simulink subsystem "Thrust_Forces_Moments"  (R2025b)
settings: Solver=VariableStepAuto  StartTime=0.0  StopTime=10.0  RelTol=1e-3
undefined symbols (not defined in the file): NumberOfEngines, phi_T, psi_T, R_n, Rho0, T_Max0, x_T_in, y_T_in, y_T_out, z_T_in, z_T_out
settings Model: Creator=cdriggs  LastModifiedBy=Ky Bui

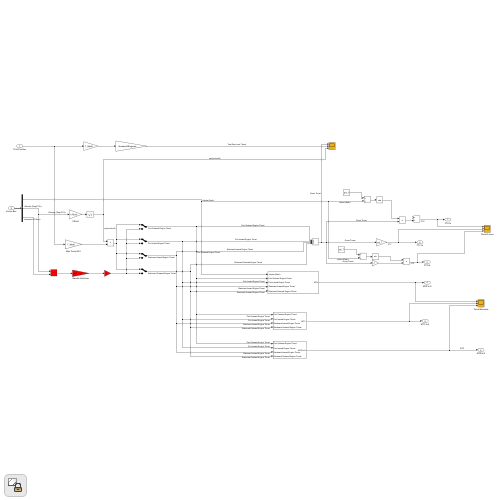
[thumbnail: Simulink's stored preview of the top-level diagram]
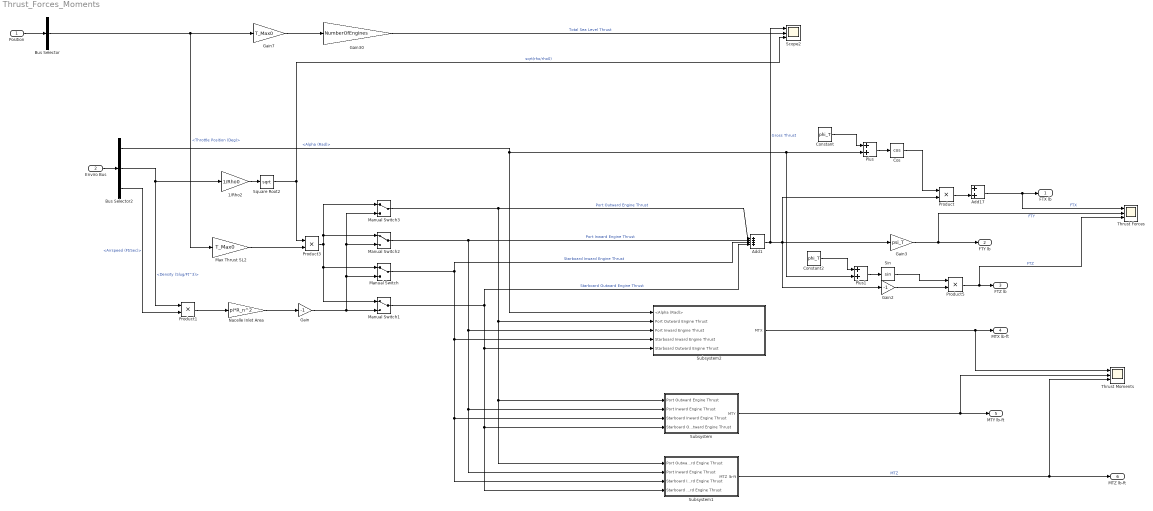
== system Thrust_Forces_Moments ==
  Position : Inport
  Enviro Bus : Inport  Port=2
  1/Rho2 : Gain  Gain=1/Rho0
  Add1 : Sum  Inputs=++++
  Add17 : Sum
  Bus Selector : BusSelector  OutputSignals=Throttle Position (Deg)
  Bus Selector2 : BusSelector  OutputSignals=Aero angles.Alpha (Rad),Density (Slug/Ft^3),Airspeed (Ft/Sec)
  Constant : Constant  Value=phi_T
  Constant2 : Constant  Value=phi_T
  Cos : Trigonometry  Operator=cos
  Gain : Gain  Gain=-1
  Gain2 : Gain  Gain=-1
  Gain3 : Gain  Gain=psi_T
  Gain30 : Gain  Gain=NumberOfEngines
  Gain7 : Gain  Gain=T_Max0
  Manual Switch{,1..3} (4 alike) : ManualSwitch
  Max Thrust SL2 : Gain  Gain=T_Max0
  Nacelle Inlet Area : Gain  Gain=pi*R_n^2
  Plus : Sum
  Plus1 : Sum
  Product{,1,3,5} (4 alike) : Product
  Scope2 : Scope  NumInputPorts=3
      settings: ActiveDisplayYMinimum=62520.103031363164  ActiveDisplayYMaximum=69799.500358108562  DataLoggingVariableName=ScopeData11
  Sin : Trigonometry
  Square Root2 : Sqrt
  Subsystem : Subsystem
  Subsystem1 : Subsystem
  Subsystem2 : Subsystem
  Thrust Forces : Scope  NumInputPorts=3
      settings: ActiveDisplayYMinimum=-15674.497725695244  ActiveDisplayYMaximum=81341.997508548971  DataLoggingVariableName=ScopeData4
  Thrust Moments : Scope  NumInputPorts=3
      settings: ActiveDisplayYMinimum=-5421.00895528758  ActiveDisplayYMaximum=48789.080597588152  DataLoggingVariableName=ScopeData5
  FTX lb : Outport
  FTY lb : Outport  Port=2
  FTZ lb : Outport  Port=3
  MTX lb-ft : Outport  Port=4
  MTY lb-ft : Outport  Port=5
  MTZ lb-ft : Outport  Port=6
  wires:
  Bus Selector2/1 -> Plus1/2, Plus/2, Subsystem2/1(<Alpha (Rad)>)  "<Alpha (Rad)>"
  Bus Selector2/2 -> 1/Rho2/1, Product1/1  "<Density (Slug/Ft^3)>"
  Add1/1 -> Scope2/1, Gain3/1, Product/2, Gain2/1  "Gross Thrust"
  Manual Switch3/1 -> Add1/1, Subsystem/1(Port Outward Engine Thrust), Subsystem1/1(Port Outward Engine Thrust), Subsystem2/2(Port Outward Engine Thrust)  "Port Outward Engine Thrust"
  Product/1 -> Add17/2
  Product3/1 -> Manual Switch3/1, Manual Switch2/1, Manual Switch1/1, Manual Switch/1
  Gain2/1 -> Product5/2
  Cos/1 -> Product/1
  Subsystem1/1(MTZ lb-ft) -> Thrust Moments/3, MTZ lb-ft/1  "MTZ"
  Constant/1 -> Plus/1
  Gain3/1 -> FTY lb/1, Thrust Forces/2  "FTY"
  Manual Switch/1 -> Subsystem2/4(Starboard Inward Engine Thrust), Subsystem/3(Starboard Inward Engine Thrust), Subsystem1/3(Starboard Inward Engine Thrust), Add1/3  "Starboard Inward Engine Thrust"
  Manual Switch2/1 -> Add1/2, Subsystem/2(Port Inward Engine Thrust), Subsystem1/2(Port Inward Engine Thrust), Subsystem2/3(Port Inward Engine Thrust)  "Port Inward Engine Thrust"
  Enviro Bus/1 -> Bus Selector2/1
  Constant2/1 -> Plus1/1
  Max Thrust SL2/1 -> Product3/2
  Manual Switch1/1 -> Subsystem2/5(Starboard Outward Engine Thrust), Subsystem/4(Starboard Outward Engine Thrust), Subsystem1/4(Starboard Outward Engine Thrust), Add1/4  "Starboard Outward Engine Thrust"
  Sin/1 -> Product5/1
  1/Rho2/1 -> Square Root2/1
  Add17/1 -> FTX lb/1, Thrust Forces/1  "FTX"
  Gain30/1 -> Scope2/2  "Total Sea Level Thrust"
  Plus1/1 -> Sin/1
  Square Root2/1 -> Product3/1, Scope2/3  "sqrt(rho/rho0)"
  Gain7/1 -> Gain30/1
  Product5/1 -> FTZ lb/1, Thrust Forces/3  "FTZ"
  Plus/1 -> Cos/1
  Subsystem/1(MTY) -> Thrust Moments/2, MTY lb-ft/1
  Subsystem2/1(MTX) -> MTX lb-ft/1, Thrust Moments/1
  Bus Selector2/3 -> Product1/2  "<Airspeed (Ft/Sec)>"
  Nacelle Inlet Area/1 -> Gain/1
  Product1/1 -> Nacelle Inlet Area/1
  Gain/1 -> Manual Switch3/2, Manual Switch2/2, Manual Switch/2, Manual Switch1/2
  Position/1 -> Bus Selector/1
  Bus Selector/1 -> Gain7/1, Max Thrust SL2/1  "<Throttle Position (Deg)>"

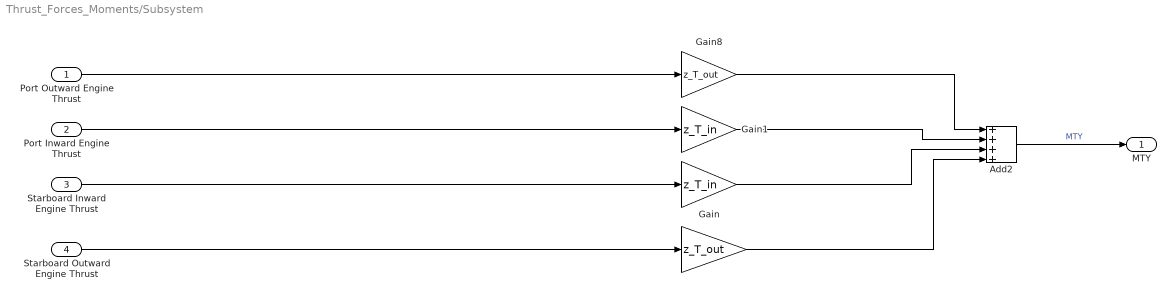
== system Thrust_Forces_Moments/Subsystem ==
  Port Outward Engine Thrust : Inport
  Port Inward Engine Thrust : Inport  Port=2
  Starboard Inward Engine Thrust : Inport  Port=3
  Starboard Outward Engine Thrust : Inport  Port=4
  " " : Gain  Gain=z_T_out
  Add2 : Sum  Inputs=++++
  Gain : Gain  Gain=z_T_in
  Gain1 : Gain  Gain=z_T_in
  Gain8 : Gain  Gain=z_T_out
  MTY : Outport
  wires:
  Port Outward Engine Thrust/1 -> Gain8/1
  Starboard Outward Engine Thrust/1 -> " "/1
  " "/1 -> Add2/4
  Starboard Inward Engine Thrust/1 -> Gain/1
  Port Inward Engine Thrust/1 -> Gain1/1
  Gain1/1 -> Add2/2
  Add2/1 -> MTY/1  "MTY"
  Gain/1 -> Add2/3
  Gain8/1 -> Add2/1

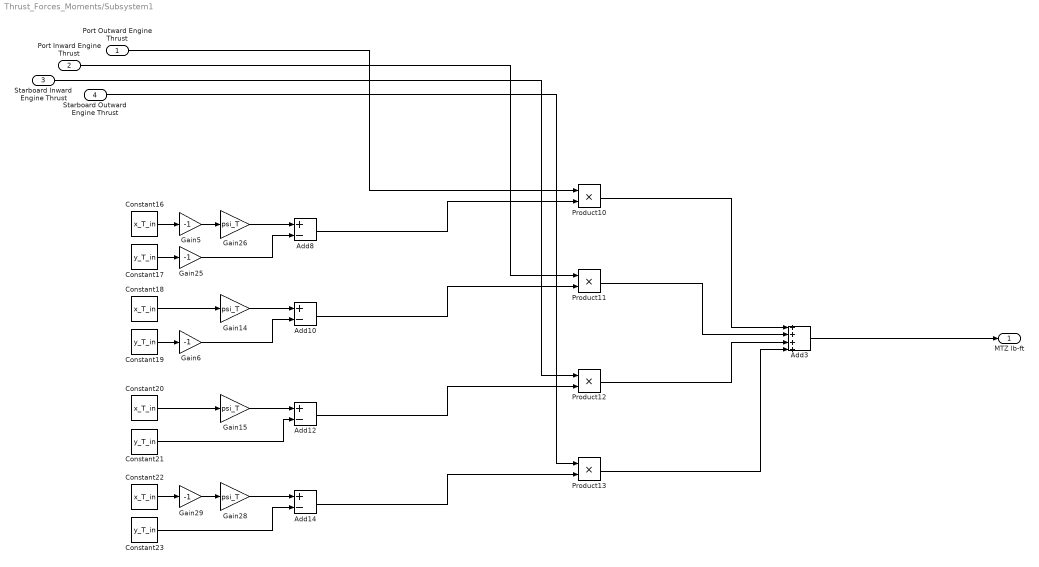
== system Thrust_Forces_Moments/Subsystem1 ==
  Port Outward Engine Thrust : Inport
  Port Inward Engine Thrust : Inport  Port=2
  Starboard Inward Engine Thrust : Inport  Port=3
  Starboard Outward Engine Thrust : Inport  Port=4
  Add{8,10,12,14} (4 alike) : Sum  Inputs=+-
  Add3 : Sum  Inputs=++++
  Constant{16,18,20,22} (4 alike) : Constant  Value=x_T_in
  Constant{17,19,21,23} (4 alike) : Constant  Value=y_T_in
  Gain{14..15,26,28} (4 alike) : Gain  Gain=psi_T
  Gain{5..6,25,29} (4 alike) : Gain  Gain=-1
  Product{10..13} (4 alike) : Product
  MTZ lb-ft : Outport
  wires:
  Gain25/1 -> Add8/2
  Constant22/1 -> Gain29/1
  Add14/1 -> Product13/2
  Starboard Inward Engine Thrust/1 -> Product12/1
  Gain15/1 -> Add12/1
  Constant20/1 -> Gain15/1
  Gain5/1 -> Gain26/1
  Gain29/1 -> Gain28/1
  Constant23/1 -> Add14/2
  Constant17/1 -> Gain25/1
  Add3/1 -> MTZ lb-ft/1
  Gain26/1 -> Add8/1
  Gain14/1 -> Add10/1
  Constant21/1 -> Add12/2
  Gain28/1 -> Add14/1
  Starboard Outward Engine Thrust/1 -> Product13/1
  Product10/1 -> Add3/1
  Constant16/1 -> Gain5/1
  Add12/1 -> Product12/2
  Port Inward Engine Thrust/1 -> Product11/1
  Port Outward Engine Thrust/1 -> Product10/1
  Add8/1 -> Product10/2
  Constant19/1 -> Gain6/1
  Product11/1 -> Add3/2
  Add10/1 -> Product11/2
  Product13/1 -> Add3/4
  Gain6/1 -> Add10/2
  Constant18/1 -> Gain14/1
  Product12/1 -> Add3/3

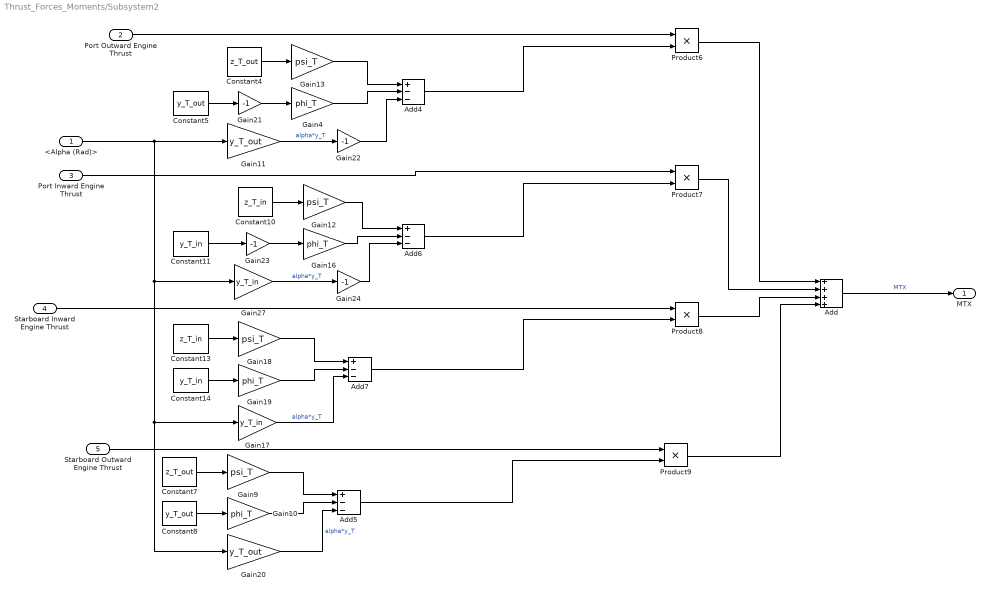
== system Thrust_Forces_Moments/Subsystem2 ==
  <Alpha (Rad)> : Inport
  Port Outward Engine Thrust : Inport  Port=2
  Port Inward Engine Thrust : Inport  Port=3
  Starboard Inward Engine Thrust : Inport  Port=4
  Starboard Outward Engine Thrust : Inport  Port=5
  Add : Sum  Inputs=++++
  Add{4..7} (4 alike) : Sum  Inputs=+--
  Constant10 : Constant  Value=z_T_in
  Constant11 : Constant  Value=y_T_in
  Constant13 : Constant  Value=z_T_in
  Constant14 : Constant  Value=y_T_in
  Constant4 : Constant  Value=z_T_out
  Constant5 : Constant  Value=y_T_out
  Constant7 : Constant  Value=z_T_out
  Constant8 : Constant  Value=y_T_out
  Gain{4,10,16,19} (4 alike) : Gain  Gain=phi_T
  Gain11 : Gain  Gain=y_T_out
  Gain{9,12..13,18} (4 alike) : Gain  Gain=psi_T
  Gain17 : Gain  Gain=y_T_in
  Gain20 : Gain  Gain=y_T_out
  Gain{21..24} (4 alike) : Gain  Gain=-1
  Gain27 : Gain  Gain=y_T_in
  Product{6..9} (4 alike) : Product
  MTX : Outport
  wires:
  Product8/1 -> Add/3
  Gain16/1 -> Add6/2
  Gain13/1 -> Add4/1
  Product6/1 -> Add/1
  Gain27/1 -> Gain24/1  "alpha*y_T"
  Gain23/1 -> Gain16/1
  Constant10/1 -> Gain12/1
  Gain24/1 -> Add6/3
  Gain9/1 -> Add5/1
  Gain12/1 -> Add6/1
  Constant11/1 -> Gain23/1
  Constant14/1 -> Gain19/1
  Port Outward Engine Thrust/1 -> Product6/1
  Add7/1 -> Product8/2
  Port Inward Engine Thrust/1 -> Product7/1
  Constant13/1 -> Gain18/1
  Gain19/1 -> Add7/2
  Constant7/1 -> Gain9/1
  Gain11/1 -> Gain22/1  "alpha*y_T"
  Starboard Inward Engine Thrust/1 -> Product8/1
  <Alpha (Rad)>/1 -> Gain11/1, Gain27/1, Gain17/1, Gain20/1
  Add6/1 -> Product7/2
  Product7/1 -> Add/2
  Add5/1 -> Product9/2
  Constant4/1 -> Gain13/1
  Constant5/1 -> Gain21/1
  Gain21/1 -> Gain4/1
  Add/1 -> MTX/1  "MTX"
  Add4/1 -> Product6/2
  Product9/1 -> Add/4
  Gain20/1 -> Add5/3  "alpha*y_T"
  Gain22/1 -> Add4/3
  Gain4/1 -> Add4/2
  Gain10/1 -> Add5/2
  Gain18/1 -> Add7/1
  Gain17/1 -> Add7/3  "alpha*y_T"
  Constant8/1 -> Gain10/1
  Starboard Outward Engine Thrust/1 -> Product9/1
